simulink model "FOC_sensored"  (R2026a)
settings: Solver=VariableStepAuto  StopTime=0.5  MaxStep=1e-4  RelTol=1e-4
values from neighbouring files (symbols this model uses):
  Encoder_resolution = 4000    [FOC_sensored_script.m]
  In = 1    [FOC_sensored_script.m]
  J = 0.1e-4    (= 1e-05)    [FOC_sensored_script.m]
  Kr_cont_current = (2*omega_n*tau_q*zeta - 1) / K_q    [FOC_sensored_script.m]
  Kr_cont_speed = (2*omega_n_speed*tau_w*zeta_speed - 1) / K_w    [FOC_sensored_script.m]
  Kr_direct_back_current = (1-delta2*exp(Ts_current/tau_q)) / (K_q*(exp(Ts_current/tau_q)-1))    [FOC_sensored_script.m]
  Kr_direct_back_speed = (1-delta2*exp(Ts_speed/tau_w)) / (K_w*(exp(Ts_speed/tau_w)-1))    [FOC_sensored_script.m]
  Kr_direct_forw_current = (1+(1+delta1)*exp(Ts_current/tau_q)) / (K_q*(exp(Ts_current/tau_q)-1))    [FOC_sensored_script.m]
  Kr_direct_tustin_current = (2-exp(Ts_current/tau_q)*(delta2-delta1-1)) / (2*K_q*(exp(Ts_current/tau_q)-1))    [FOC_sensored_script.m]
  Kr_direct_tustin_speed = (2-exp(Ts_speed/tau_w)*(delta2-delta1-1)) / (2*K_w*(exp(Ts_speed/tau_w)-1))    [FOC_sensored_script.m]
  Ls = 330e-6/2    (= 0.000165)    [FOC_sensored_script.m]
  Mn = Pn/wn    [FOC_sensored_script.m]
  nn = ns/pp    (= 6000)    [FOC_sensored_script.m]
  pp = (60*fs)/ns    (= 4)    [FOC_sensored_script.m]
  Psir = 0.0064    [FOC_sensored_script.m]
  T_speed_feedback = 0.0005    [FOC_sensored_script.m]
  Ti_cont_current = (2*omega_n*tau_q*zeta - 1) / (tau_q * omega_n^2)    [FOC_sensored_script.m]
  Ti_cont_speed = (2*omega_n_speed*tau_w*zeta_speed - 1) / (tau_w * omega_n_speed^2)    [FOC_sensored_script.m]
  Ti_direct_back_current = Ts_current * (exp(-Ts_current/tau_q)-delta2) / (1+delta1+delta2)    [FOC_sensored_script.m]
  Ti_direct_back_speed = Ts_speed * (exp(-Ts_speed/tau_w)-delta2) / (1+delta1+delta2)    [FOC_sensored_script.m]
  Ti_direct_forw_current = Ts_current * (1+delta1+exp(-Ts_current/tau_q)) / (1+delta1+delta2)    [FOC_sensored_script.m]
  Ti_direct_forw_speed = Ts_speed * (1+delta1+exp(-Ts_speed/tau_w)) / (1+delta1+delta2)    [FOC_sensored_script.m]
  Ti_direct_tustin_current = Ts_current*(2*exp(-Ts_current/tau_q)+delta1-delta2+1) / (2*(1+delta1+delta2))    [FOC_sensored_script.m]
  Ti_direct_tustin_speed = Ts_speed*(2*exp(-Ts_speed/tau_w)+delta1-delta2+1) / (2*(1+delta1+delta2))    [FOC_sensored_script.m]
  Ts_current = 100e-6    (= 0.0001)    [FOC_sensored_script.m]
  Udc = 24    [FOC_sensored_script.m]
undefined symbols (not defined in the file or in its folder): Ld, Lq
libraries: fl_lib x48, nesl_utility x42, ee_lib x18, eeTransforms x12
(part 3 of 3)

== system FOC_sensored/PWM inverter7 ==
  ud_ref : Inport
  uq_ref : Inport  Port=2
  theta_e_mj : Inport  Port=3
  Constant1 : Constant  Value=0  SampleTime=-1
  Gain : Gain
  Gain1 : Gain
  Mux2 : Mux  Inputs=2
  Mux3 : Mux  Inputs=2
  Scope : Scope  NumInputPorts=2
      settings: ActiveDisplayYMinimum=-5.00439749396322  ActiveDisplayYMaximum=16.069405098335697
  Zero-Order Hold1 : ZeroOrderHold  SampleTime=Ts_current
  dq->abc : eeTransforms/Inverse Park Transform  AxisAlignment=D-axis  PowerInvariant=off
  u_abc* : Outport  VectorParamsAs1DForOutWhenUnconnected=off
  wires:
  Constant1/1 -> Mux2/2
  Mux2/1 -> dq->abc/1
  Mux3/1 -> Mux2/1
  theta_e_mj/1 -> dq->abc/2
  dq->abc/1 -> Zero-Order Hold1/1
  ud_ref/1 -> Gain/1
  uq_ref/1 -> Gain1/1
  Gain/1 -> Scope/1, Mux3/1
  Gain1/1 -> Scope/2, Mux3/2
  Zero-Order Hold1/1 -> u_abc*/1

== matlab function FOC_sensored/Low-Pass Filter Speed ==
  data: x input; y output; y_prev input; y_prev_out output; x_prev input; x_prev_out output; fc input; TS input
function [y, y_prev_out, x_prev_out] = fcn(x, y_prev, x_prev, fc, TS)


%% Convert to rad/s
omega_c = 2 * pi * fc;

%% Tustin coefficients
b =  omega_c / (2/TS + omega_c);
a = (omega_c - 2/TS) / (2/TS + omega_c);

%% Output
y = b * (x + x_prev) - a * y_prev;

%% State outputs — two separate scalars
y_prev_out = y;
x_prev_out = x;

end

== matlab function FOC_sensored/Low-Pass Filter Current ==
  data: x input; y output; y_prev input; y_prev_out output; x_prev input; x_prev_out output; fc input; TS input
function [y, y_prev_out, x_prev_out] = fcn(x, y_prev, x_prev, fc, TS)



%% Convert to rad/s
omega_c = 2 * pi * fc;

%% Tustin coefficients
b =  omega_c / (2/TS + omega_c);
a = (omega_c - 2/TS) / (2/TS + omega_c);

%% Output
y = b * (x + x_prev) - a * y_prev;

%% State outputs — two separate scalars
y_prev_out = y;
x_prev_out = x;

end

== matlab function FOC_sensored/Low-Pass Filter Speed Ref ==
  data: x input; y output; y_prev input; y_prev_out output; x_prev input; x_prev_out output; fc input; TS input
function [y, y_prev_out, x_prev_out] = fcn(x, y_prev, x_prev, fc, TS)

%% Convert to rad/s
omega_c = 2 * pi * fc;

%% Tustin coefficients
b =  omega_c / (2/TS + omega_c);
a = (omega_c - 2/TS) / (2/TS + omega_c);

%% Output
y = b * (x + x_prev) - a * y_prev;

%% State outputs — two separate scalars
y_prev_out = y;
x_prev_out = x;

end

== matlab function FOC_sensored/Diskretni regulator brzine1/PI-speed_controller ==
  data: speed_ref input; is_ref output; speed input; error_prev input; integrator_state input; error_out output; vd_state_out output; speed_ref_sat output; MAX_RPM input; K_P_speed input; K_I_speed input; TS input; IS_REF_LIMIT input
function [is_ref, error_out, vd_state_out,speed_ref_sat] = ...
          fcn(speed_ref, speed, error_prev, integrator_state, MAX_RPM, K_P_speed, K_I_speed, TS, IS_REF_LIMIT)



%% Saturate speed reference
if speed_ref > MAX_RPM
    speed_ref_sat = MAX_RPM;
elseif speed_ref < -MAX_RPM
    speed_ref_sat = -MAX_RPM;
else
    speed_ref_sat = speed_ref;
end

%% Error
error_curr = speed_ref_sat - speed;

%% --- Tustin (bilinear) PI ---
%
%  Continuous PI:   u(s) = Kp * e(s) + Ki/s * e(s)
%
%  Tustin:  integrator  1/s  ->  T/2 * (z+1)/(z-1)
%
%  Incremental form:
%    u[k] = u[k-1] + Kp*(e[k] - e[k-1]) + Ki*T/2*(e[k] + e[k-1])

is_ref_raw = integrator_state ...
           + K_P_speed * (error_curr - error_prev) ...
           + K_I_speed * (TS / 2.0) * (error_curr + error_prev);

%% Saturate is_ref (anti-windup: clamp before feeding state back)
if is_ref_raw > IS_REF_LIMIT
    is_ref = IS_REF_LIMIT;
elseif is_ref_raw < -IS_REF_LIMIT
    is_ref = -IS_REF_LIMIT;
else
    is_ref = is_ref_raw;
end

%% State outputs → Unit Delays → next step inputs
error_out      = error_curr;   % → Unit Delay → error_prev
vd_state_out   = is_ref;       % → Unit Delay → integrator_state (clamped = anti-windup)

end

== matlab function FOC_sensored/Diskretni regulatori struje2/PI-controller ==
  data: error_id input; error_iq input; id input; iq input; we_prev input; vd output; vq output; vd_state_in input; vq_state_in input; error_id_prev input; error_iq_prev input; vd_state_out output; vq_state_out output; error_id_out output; error_iq_out output; ff_id_prev input; ff_iq_prev input; ff_id_out output; ff_iq_out output; K_P_current input; K_I_current input; TS input; L_Q input; L_D input; PHI_PM input; CURRENT_CONTROL_LIMIT input
function [vd, vq, vd_state_out, vq_state_out, ...
          error_id_out, error_iq_out, ff_id_out, ff_iq_out] = ...
          fcn(error_id, error_iq, id, iq, we_prev, ...
              vd_state_in, vq_state_in, ...
              error_id_prev, error_iq_prev, ...
              ff_id_prev, ff_iq_prev, K_P_current, K_I_current, TS, L_Q, L_D, PHI_PM, CURRENT_CONTROL_LIMIT)


%% Feedforward — using delayed we to break algebraic loop
ff_id = -iq * L_Q * we_prev;
ff_iq =  id * L_D * we_prev + PHI_PM * we_prev;

%% Tustin PI + FF delta
vd_ = vd_state_in ...
    + K_P_current * (error_id - error_id_prev) ...
    + K_I_current * (TS / 2) * (error_id + error_id_prev) ...
    + (ff_id - ff_id_prev);

vq_ = vq_state_in ...
    + K_P_current * (error_iq - error_iq_prev) ...
    + K_I_current * (TS / 2) * (error_iq + error_iq_prev) ...
    + (ff_iq - ff_iq_prev);

%% Circle clamp
voltage_magnitude = sqrt(vd_^2 + vq_^2);
if voltage_magnitude > CURRENT_CONTROL_LIMIT
    scale = CURRENT_CONTROL_LIMIT / voltage_magnitude;
    vd = vd_ * scale;
    vq = vq_ * scale;
else
    vd = vd_;
    vq = vq_;
end

%% State outputs
vd_state_out = vd;
vq_state_out = vq;
error_id_out = error_id;
error_iq_out = error_iq;
ff_id_out    = ff_id;      % → Unit Delay → ff_id_prev
ff_iq_out    = ff_iq;      % → Unit Delay → ff_iq_prev

end

== matlab function FOC_sensored/Encoder1 ==
  data: angle input; theta_e output; omega_e output; angle_prev input; q_angle output; N input; dt input; pole_pairs input
function [theta_e, omega_e, q_angle] = fcn(angle, angle_prev, N, dt, pole_pairs)

%% Quantize current angle (simulate encoder resolution)
raw_count   = angle * (N / (2*pi));
counts      = floor(raw_count + 0.5);
q_angle     = counts * (2*pi / N);

%% Quantize previous angle the same way
raw_count_prev = angle_prev * (N / (2*pi));
counts_prev    = floor(raw_count_prev + 0.5);
q_angle_prev   = counts_prev * (2*pi / N);

%% Mechanical angular velocity (handle wrap-around)
delta = q_angle - q_angle_prev;

% Unwrap: if jump > pi, crossed zero boundary
if delta > pi
    delta = delta - 2*pi;
elseif delta < -pi
    delta = delta + 2*pi;
end

omega_m = delta / dt;       % mechanical rad/s

%% Convert to electrical quantities
theta_e = mod(q_angle, 2*pi);   % electrical angle [0, 2pi]
omega_e = omega_m;               % electrical rad/s

end

== matlab function FOC_sensored/Low-Pass Filter Current1 ==
  data: x input; y output; y_prev input; y_prev_out output; x_prev input; x_prev_out output; fc input; TS input
function [y, y_prev_out, x_prev_out] = fcn(x, y_prev, x_prev, fc, TS)



%% Convert to rad/s
omega_c = 2 * pi * fc;

%% Tustin coefficients
b =  omega_c / (2/TS + omega_c);
a = (omega_c - 2/TS) / (2/TS + omega_c);

%% Output
y = b * (x + x_prev) - a * y_prev;

%% State outputs — two separate scalars
y_prev_out = y;
x_prev_out = x;

end

== matlab function FOC_sensored/Low-Pass Filter Speed Ref1 ==
  data: x input; y output; y_prev input; y_prev_out output; x_prev input; x_prev_out output; fc input; TS input
function [y, y_prev_out, x_prev_out] = fcn(x, y_prev, x_prev, fc, TS)

%% Convert to rad/s
omega_c = 2 * pi * fc;

%% Tustin coefficients
b =  omega_c / (2/TS + omega_c);
a = (omega_c - 2/TS) / (2/TS + omega_c);

%% Output
y = b * (x + x_prev) - a * y_prev;

%% State outputs — two separate scalars
y_prev_out = y;
x_prev_out = x;

end

== matlab function FOC_sensored/Low-Pass Filter Speed1 ==
  data: x input; y output; y_prev input; y_prev_out output; x_prev input; x_prev_out output; fc input; TS input
function [y, y_prev_out, x_prev_out] = fcn(x, y_prev, x_prev, fc, TS)


%% Convert to rad/s
omega_c = 2 * pi * fc;

%% Tustin coefficients
b =  omega_c / (2/TS + omega_c);
a = (omega_c - 2/TS) / (2/TS + omega_c);

%% Output
y = b * (x + x_prev) - a * y_prev;

%% State outputs — two separate scalars
y_prev_out = y;
x_prev_out = x;

end

== matlab function FOC_sensored/Diskretni regulator brzine2/PI-speed_controller ==
  data: speed_ref input; is_ref output; vd_state_out output; speed input; vd_state_in input; error_prev input; error_out output; MAX_RPM input; K_P_speed input; K_I_speed input; TS input; IS_REF_LIMIT input
function [is_ref, vd_state_out, error_out] = ...
          fcn(speed_ref, speed, vd_state_in, error_prev, MAX_RPM, K_P_speed, K_I_speed, TS, IS_REF_LIMIT)


%% Saturate speed reference
if speed_ref > MAX_RPM
    speed_ref_sat = MAX_RPM;
elseif speed_ref < -MAX_RPM
    speed_ref_sat = -MAX_RPM;
else
    speed_ref_sat = speed_ref;
end

%% Error
error_curr = speed_ref_sat - speed;

%% --- Backward Euler PI ---
%
%  u[k] = u[k-1] + Kp*(e[k] - e[k-1]) + Ki*TS*e[k]

is_ref_raw = vd_state_in ...
           + K_P_speed * (error_curr - error_prev) ...
           + K_I_speed * TS * error_curr;

%% Saturate is_ref
if is_ref_raw > IS_REF_LIMIT
    is_ref = IS_REF_LIMIT;
elseif is_ref_raw < -IS_REF_LIMIT
    is_ref = -IS_REF_LIMIT;
else
    is_ref = is_ref_raw;
end

%% Conditional anti-windup — freeze integrator when saturated
saturated = (is_ref_raw > IS_REF_LIMIT && error_curr > 0) || ...
            (is_ref_raw < -IS_REF_LIMIT && error_curr < 0);

if saturated
    vd_state_out = vd_state_in;   % freeze
else
    vd_state_out = is_ref;
end

%% State output
error_out = error_curr;

end

== matlab function FOC_sensored/Diskretni regulatori struje1/PI-controller ==
  data: error_id input; error_iq input; vd output; vq output; vd_state_in input; vq_state_in input; vd_state_out output; vq_state_out output; error_id_prev input; error_iq_prev input; error_id_out output; error_iq_out output; K_P_current input; K_I_current input; TS input; CURRENT_CONTROL_LIMIT input
function [vd, vq, vd_state_out, vq_state_out, ...
          error_id_out, error_iq_out] = ...
          fcn(error_id, error_iq, ...
              vd_state_in, vq_state_in, ...
              error_id_prev, error_iq_prev, K_P_current, K_I_current, TS, CURRENT_CONTROL_LIMIT)


%% Backward Euler PI — incremental form
%
%  u[k] = u[k-1] + Kp*(e[k] - e[k-1]) + Ki*TS*e[k]

vd_ = vd_state_in ...
    + K_P_current * (error_id - error_id_prev) ...
    + K_I_current * TS * error_id;

vq_ = vq_state_in ...
    + K_P_current * (error_iq - error_iq_prev) ...
    + K_I_current * TS * error_iq;

%% Circle clamp
voltage_magnitude = sqrt(vd_^2 + vq_^2);
if voltage_magnitude > CURRENT_CONTROL_LIMIT
    scale = CURRENT_CONTROL_LIMIT / voltage_magnitude;
    vd = vd_ * scale;
    vq = vq_ * scale;
else
    vd = vd_;
    vq = vq_;
end

%% State outputs
vd_state_out  = vd;     % anti-windup: feed back clamped value
vq_state_out  = vq;
error_id_out  = error_id;
error_iq_out  = error_iq;

end

== matlab function FOC_sensored/Encoder2 ==
  data: angle input; theta_e output; omega_e output; angle_prev input; q_angle output; N input; dt input; pole_pairs input
function [theta_e, omega_e, q_angle] = fcn(angle, angle_prev, N, dt, pole_pairs)

%% Quantize current angle (simulate encoder resolution)
raw_count   = angle * (N / (2*pi));
counts      = floor(raw_count + 0.5);
q_angle     = counts * (2*pi / N);

%% Quantize previous angle the same way
raw_count_prev = angle_prev * (N / (2*pi));
counts_prev    = floor(raw_count_prev + 0.5);
q_angle_prev   = counts_prev * (2*pi / N);

%% Mechanical angular velocity (handle wrap-around)
delta = q_angle - q_angle_prev;

% Unwrap: if jump > pi, crossed zero boundary
if delta > pi
    delta = delta - 2*pi;
elseif delta < -pi
    delta = delta + 2*pi;
end

omega_m = delta / dt;       % mechanical rad/s

%% Convert to electrical quantities
theta_e = mod(q_angle, 2*pi);   % electrical angle [0, 2pi]
omega_e = omega_m;               % electrical rad/s

end

== matlab function FOC_sensored/Low-Pass Filter Current2 ==
  data: x input; y output; y_prev input; y_prev_out output; fc input; TS input
function [y, y_prev_out] = fcn(x, y_prev, fc, TS)


%% Convert to rad/s
omega_c = 2 * pi * fc;

%% Backward Euler discretization of H(s) = omega_c / (s + omega_c)
%
%  Backward Euler:  s -> (z-1)/(TS*z)
%
%  H(z) = omega_c / ((z-1)/(TS*z) + omega_c)
%
%  Multiply numerator and denominator by TS*z:
%
%  H(z) = omega_c*TS*z / ((z-1) + omega_c*TS*z)
%
%  Collecting z terms:
%
%  numerator:   omega_c*TS * z
%  denominator: (1 + omega_c*TS)*z - 1
%
%  Divide by (1 + omega_c*TS):
%
%  b = omega_c*TS / (1 + omega_c*TS)
%  a = 1 / (1 + omega_c*TS)
%
%  Difference equation:
%  y[k] = b*x[k] + a*y[k-1]

%% Precompute coefficients
b = (omega_c*TS) / (1 + omega_c*TS);
a = 1 / (1 + omega_c*TS);

%% Output — note: Backward Euler only needs y_prev, not x_prev
y = b * x + a * y_prev;

%% State outputs
y_prev_out = y;

end

== matlab function FOC_sensored/Low-Pass Filter Speed Ref2 ==
  data: x input; y output; y_prev input; y_prev_out output; fc input; TS input
function [y, y_prev_out] = fcn(x, y_prev, fc, TS)


%% Convert to rad/s
omega_c = 2 * pi * fc;

%% Backward Euler discretization of H(s) = omega_c / (s + omega_c)
%
%  Backward Euler:  s -> (z-1)/(TS*z)
%
%  H(z) = omega_c / ((z-1)/(TS*z) + omega_c)
%
%  Multiply numerator and denominator by TS*z:
%
%  H(z) = omega_c*TS*z / ((z-1) + omega_c*TS*z)
%
%  Collecting z terms:
%
%  numerator:   omega_c*TS * z
%  denominator: (1 + omega_c*TS)*z - 1
%
%  Divide by (1 + omega_c*TS):
%
%  b = omega_c*TS / (1 + omega_c*TS)
%  a = 1 / (1 + omega_c*TS)
%
%  Difference equation:
%  y[k] = b*x[k] + a*y[k-1]

%% Precompute coefficients
b = (omega_c*TS) / (1 + omega_c*TS);
a = 1 / (1 + omega_c*TS);

%% Output — note: Backward Euler only needs y_prev, not x_prev
y = b * x + a * y_prev;

%% State outputs
y_prev_out = y;

end

== matlab function FOC_sensored/Low-Pass Filter Speed2 ==
  data: x input; y output; y_prev input; y_prev_out output; fc input; TS input
function [y, y_prev_out] = fcn(x, y_prev, fc, TS)


%% Convert to rad/s
omega_c = 2 * pi * fc;

%% Backward Euler discretization of H(s) = omega_c / (s + omega_c)
%
%  Backward Euler:  s -> (z-1)/(TS*z)
%
%  H(z) = omega_c / ((z-1)/(TS*z) + omega_c)
%
%  Multiply numerator and denominator by TS*z:
%
%  H(z) = omega_c*TS*z / ((z-1) + omega_c*TS*z)
%
%  Collecting z terms:
%
%  numerator:   omega_c*TS * z
%  denominator: (1 + omega_c*TS)*z - 1
%
%  Divide by (1 + omega_c*TS):
%
%  b = omega_c*TS / (1 + omega_c*TS)
%  a = 1 / (1 + omega_c*TS)
%
%  Difference equation:
%  y[k] = b*x[k] + a*y[k-1]

%% Precompute coefficients
b = (omega_c*TS) / (1 + omega_c*TS);
a = 1 / (1 + omega_c*TS);

%% Output — note: Backward Euler only needs y_prev, not x_prev
y = b * x + a * y_prev;

%% State outputs
y_prev_out = y;

end

== matlab function FOC_sensored/Diskretni regulator brzine3/PI-speed_controller ==
  data: speed_ref input; is_ref output; speed input; error_prev input; integrator_state input; error_out output; vd_state_out output; speed_ref_sat output; MAX_RPM input; K_P_speed input; K_I_speed input; TS input; IS_REF_LIMIT input
function [is_ref, error_out, vd_state_out,speed_ref_sat] = ...
          fcn(speed_ref, speed, error_prev, integrator_state, MAX_RPM, K_P_speed, K_I_speed, TS, IS_REF_LIMIT)



%% Saturate speed reference
if speed_ref > MAX_RPM
    speed_ref_sat = MAX_RPM;
elseif speed_ref < -MAX_RPM
    speed_ref_sat = -MAX_RPM;
else
    speed_ref_sat = speed_ref;
end

%% Error
error_curr = speed_ref_sat - speed;

%% --- Tustin (bilinear) PI ---
%
%  Continuous PI:   u(s) = Kp * e(s) + Ki/s * e(s)
%
%  Tustin:  integrator  1/s  ->  T/2 * (z+1)/(z-1)
%
%  Incremental form:
%    u[k] = u[k-1] + Kp*(e[k] - e[k-1]) + Ki*T/2*(e[k] + e[k-1])

is_ref_raw = integrator_state ...
           + K_P_speed * (error_curr - error_prev) ...
           + K_I_speed * (TS / 2.0) * (error_curr + error_prev);

%% Saturate is_ref (anti-windup: clamp before feeding state back)
if is_ref_raw > IS_REF_LIMIT
    is_ref = IS_REF_LIMIT;
elseif is_ref_raw < -IS_REF_LIMIT
    is_ref = -IS_REF_LIMIT;
else
    is_ref = is_ref_raw;
end

%% State outputs → Unit Delays → next step inputs
error_out      = error_curr;   % → Unit Delay → error_prev
vd_state_out   = is_ref;       % → Unit Delay → integrator_state (clamped = anti-windup)

end

== matlab function FOC_sensored/Diskretni regulatori struje3/PI-controller ==
  data: error_id input; error_iq input; id input; iq input; we_prev input; vd output; vq output; vd_state_in input; vq_state_in input; error_id_prev input; error_iq_prev input; vd_state_out output; vq_state_out output; error_id_out output; error_iq_out output; ff_id_prev input; ff_iq_prev input; ff_id_out output; ff_iq_out output; K_P_current input; K_I_current input; TS input; L_Q input; L_D input; PHI_PM input; CURRENT_CONTROL_LIMIT input
function [vd, vq, vd_state_out, vq_state_out, ...
          error_id_out, error_iq_out, ff_id_out, ff_iq_out] = ...
          fcn(error_id, error_iq, id, iq, we_prev, ...
              vd_state_in, vq_state_in, ...
              error_id_prev, error_iq_prev, ...
              ff_id_prev, ff_iq_prev, K_P_current, K_I_current, TS, L_Q, L_D, PHI_PM, CURRENT_CONTROL_LIMIT)


%% Feedforward — using delayed we to break algebraic loop
ff_id = -iq * L_Q * we_prev;
ff_iq =  id * L_D * we_prev + PHI_PM * we_prev;

%% Tustin PI + FF delta
vd_ = vd_state_in ...
    + K_P_current * (error_id - error_id_prev) ...
    + K_I_current * (TS / 2) * (error_id + error_id_prev) ...
    + (ff_id - ff_id_prev);

vq_ = vq_state_in ...
    + K_P_current * (error_iq - error_iq_prev) ...
    + K_I_current * (TS / 2) * (error_iq + error_iq_prev) ...
    + (ff_iq - ff_iq_prev);

%% Circle clamp
voltage_magnitude = sqrt(vd_^2 + vq_^2);
if voltage_magnitude > CURRENT_CONTROL_LIMIT
    scale = CURRENT_CONTROL_LIMIT / voltage_magnitude;
    vd = vd_ * scale;
    vq = vq_ * scale;
else
    vd = vd_;
    vq = vq_;
end

%% State outputs
vd_state_out = vd;
vq_state_out = vq;
error_id_out = error_id;
error_iq_out = error_iq;
ff_id_out    = ff_id;      % → Unit Delay → ff_id_prev
ff_iq_out    = ff_iq;      % → Unit Delay → ff_iq_prev

end

== matlab function FOC_sensored/Encoder3 ==
  data: angle input; theta_e output; omega_e output; angle_prev input; q_angle output; N input; dt input; pole_pairs input
function [theta_e, omega_e, q_angle] = fcn(angle, angle_prev, N, dt, pole_pairs)

%% Quantize current angle (simulate encoder resolution)
raw_count   = angle * (N / (2*pi));
counts      = floor(raw_count + 0.5);
q_angle     = counts * (2*pi / N);

%% Quantize previous angle the same way
raw_count_prev = angle_prev * (N / (2*pi));
counts_prev    = floor(raw_count_prev + 0.5);
q_angle_prev   = counts_prev * (2*pi / N);

%% Mechanical angular velocity (handle wrap-around)
delta = q_angle - q_angle_prev;

% Unwrap: if jump > pi, crossed zero boundary
if delta > pi
    delta = delta - 2*pi;
elseif delta < -pi
    delta = delta + 2*pi;
end

omega_m = delta / dt;       % mechanical rad/s

%% Convert to electrical quantities
theta_e = mod(q_angle, 2*pi);   % electrical angle [0, 2pi]
omega_e = omega_m;               % electrical rad/s

end

== matlab function FOC_sensored/Low-Pass Filter Current3 ==
  data: x input; y output; y_prev input; y_prev_out output; x_prev input; x_prev_out output; fc input; TS input
function [y, y_prev_out, x_prev_out] = fcn(x, y_prev, x_prev, fc, TS)



%% Convert to rad/s
omega_c = 2 * pi * fc;

%% Tustin coefficients
b =  omega_c / (2/TS + omega_c);
a = (omega_c - 2/TS) / (2/TS + omega_c);

%% Output
y = b * (x + x_prev) - a * y_prev;

%% State outputs — two separate scalars
y_prev_out = y;
x_prev_out = x;

end

== matlab function FOC_sensored/Low-Pass Filter Speed Ref3 ==
  data: x input; y output; y_prev input; y_prev_out output; x_prev input; x_prev_out output; fc input; TS input
function [y, y_prev_out, x_prev_out] = fcn(x, y_prev, x_prev, fc, TS)

%% Convert to rad/s
omega_c = 2 * pi * fc;

%% Tustin coefficients
b =  omega_c / (2/TS + omega_c);
a = (omega_c - 2/TS) / (2/TS + omega_c);

%% Output
y = b * (x + x_prev) - a * y_prev;

%% State outputs — two separate scalars
y_prev_out = y;
x_prev_out = x;

end

== matlab function FOC_sensored/Low-Pass Filter Speed3 ==
  data: x input; y output; y_prev input; y_prev_out output; x_prev input; x_prev_out output; fc input; TS input
function [y, y_prev_out, x_prev_out] = fcn(x, y_prev, x_prev, fc, TS)


%% Convert to rad/s
omega_c = 2 * pi * fc;

%% Tustin coefficients
b =  omega_c / (2/TS + omega_c);
a = (omega_c - 2/TS) / (2/TS + omega_c);

%% Output
y = b * (x + x_prev) - a * y_prev;

%% State outputs — two separate scalars
y_prev_out = y;
x_prev_out = x;

end

== matlab function FOC_sensored/Diskretni regulator brzine4/PI-speed_controller ==
  data: speed_ref input; is_ref output; vd_state_out output; speed input; vd_state_in input; error_prev input; error_out output; MAX_RPM input; K_P_speed input; K_I_speed input; TS input; IS_REF_LIMIT input
function [is_ref, vd_state_out, error_out] = ...
          fcn(speed_ref, speed, vd_state_in, error_prev, MAX_RPM, K_P_speed, K_I_speed, TS, IS_REF_LIMIT)


%% Saturate speed reference
if speed_ref > MAX_RPM
    speed_ref_sat = MAX_RPM;
elseif speed_ref < -MAX_RPM
    speed_ref_sat = -MAX_RPM;
else
    speed_ref_sat = speed_ref;
end

%% Error
error_curr = speed_ref_sat - speed;

%% --- Forward Euler PI ---
%
%  u[k] = u[k-1] + Kp*(e[k] - e[k-1]) + Ki*TS*e[k-1]

is_ref_raw = vd_state_in ...
           + K_P_speed * (error_curr - error_prev) ...
           + K_I_speed * TS * error_prev;

%% Saturate is_ref
if is_ref_raw > IS_REF_LIMIT
    is_ref = IS_REF_LIMIT;
elseif is_ref_raw < -IS_REF_LIMIT
    is_ref = -IS_REF_LIMIT;
else
    is_ref = is_ref_raw;
end

%% Conditional anti-windup — freeze integrator when saturated
saturated = (is_ref_raw > IS_REF_LIMIT && error_curr > 0) || ...
            (is_ref_raw < -IS_REF_LIMIT && error_curr < 0);

if saturated
    vd_state_out = vd_state_in;   % freeze
else
    vd_state_out = is_ref;
end

%% State output
error_out = error_curr;

end

== matlab function FOC_sensored/Diskretni regulatori struje4/PI-controller ==
  data: error_id input; error_iq input; vd output; vq output; vd_state_in input; vq_state_in input; vd_state_out output; vq_state_out output; error_id_prev input; error_iq_prev input; error_id_out output; error_iq_out output; K_P_current input; K_I_current input; TS input; CURRENT_CONTROL_LIMIT input
function [vd, vq, vd_state_out, vq_state_out, ...
          error_id_out, error_iq_out] = ...
          fcn(error_id, error_iq, ...
              vd_state_in, vq_state_in, ...
              error_id_prev, error_iq_prev, K_P_current, K_I_current, TS, CURRENT_CONTROL_LIMIT)


%% Forward Euler PI — incremental form
%
%  Continuous PI:  u(s) = Kp*e(s) + Ki/s * e(s)
%
%  Forward Euler integral:  integral[k] = integral[k-1] + TS*e[k-1]
%
%  Incremental form:
%    u[k] = u[k-1] + Kp*(e[k] - e[k-1]) + Ki*TS*e[k-1]
%
%  Note: integral term uses e[k-1], NOT e[k] — this is what makes
%  it "forward" (uses past error to step forward)

vd_ = vd_state_in ...
    + K_P_current * (error_id - error_id_prev) ...
    + K_I_current * TS * error_id_prev;

vq_ = vq_state_in ...
    + K_P_current * (error_iq - error_iq_prev) ...
    + K_I_current * TS * error_iq_prev;

%% Circle clamp
voltage_magnitude = sqrt(vd_^2 + vq_^2);
if voltage_magnitude > CURRENT_CONTROL_LIMIT
    scale = CURRENT_CONTROL_LIMIT / voltage_magnitude;
    vd = vd_ * scale;
    vq = vq_ * scale;
else
    vd = vd_;
    vq = vq_;
end

%% State outputs
vd_state_out  = vd;
vq_state_out  = vq;
error_id_out  = error_id;
error_iq_out  = error_iq;

end

== matlab function FOC_sensored/Encoder4 ==
  data: angle input; theta_e output; omega_e output; angle_prev input; q_angle output; N input; dt input; pole_pairs input
function [theta_e, omega_e, q_angle] = fcn(angle, angle_prev, N, dt, pole_pairs)

%% Quantize current angle (simulate encoder resolution)
raw_count   = angle * (N / (2*pi));
counts      = floor(raw_count + 0.5);
q_angle     = counts * (2*pi / N);

%% Quantize previous angle the same way
raw_count_prev = angle_prev * (N / (2*pi));
counts_prev    = floor(raw_count_prev + 0.5);
q_angle_prev   = counts_prev * (2*pi / N);

%% Mechanical angular velocity (handle wrap-around)
delta = q_angle - q_angle_prev;

% Unwrap: if jump > pi, crossed zero boundary
if delta > pi
    delta = delta - 2*pi;
elseif delta < -pi
    delta = delta + 2*pi;
end

omega_m = delta / dt;       % mechanical rad/s

%% Convert to electrical quantities
theta_e = mod(q_angle, 2*pi);   % electrical angle [0, 2pi]
omega_e = omega_m;               % electrical rad/s

end

== matlab function FOC_sensored/Low-Pass Filter Current4 ==
  data: x input; y output; y_prev input; x_prev input; y_prev_out output; fc input; TS input; x_prev_out output
function [y, y_prev_out, x_prev_out] = fcn(x, y_prev, x_prev, fc, TS)


%% Convert to rad/s
omega_c = 2 * pi * fc;

%% Forward Euler discretization of H(s) = omega_c / (s + omega_c)
%
%  Forward Euler:  s -> (z-1)/TS
%
%  H(z) = omega_c / ((z-1)/TS + omega_c)
%
%  Multiply numerator and denominator by TS:
%
%  H(z) = omega_c*TS / ((z-1) + omega_c*TS)
%
%  Collecting z terms:
%
%  numerator:   omega_c*TS
%  denominator: z + (omega_c*TS - 1)
%
%  Difference equation derivation from H(z) = Y(z)/X(z):
%
%  z*Y(z) + (omega_c*TS - 1)*Y(z) = omega_c*TS*X(z)
%  y[k+1] = (1 - omega_c*TS)*y[k] + omega_c*TS*x[k]
%
%  Shifting index back by one (k -> k-1):
%  y[k] = (1 - omega_c*TS)*y[k-1] + omega_c*TS*x[k-1]
%
%  Note: Forward Euler uses x[k-1], NOT x[k] — this is the key difference

%% Precompute coefficients
a = 1 - omega_c*TS;
b = omega_c*TS;

%% Output — uses x_prev, not x (this is what makes it "forward")
y = a * y_prev + b * x_prev;

%% State outputs
y_prev_out = y;
x_prev_out = x;

end

== matlab function FOC_sensored/Encoder ==
  data: angle input; theta_e output; omega_e output; angle_prev input; q_angle output; N input; dt input; pole_pairs input
function [theta_e, omega_e, q_angle] = fcn(angle, angle_prev, N, dt, pole_pairs)

%% Quantize current angle (simulate encoder resolution)
raw_count   = angle * (N / (2*pi));
counts      = floor(raw_count + 0.5);
q_angle     = counts * (2*pi / N);

%% Quantize previous angle the same way
raw_count_prev = angle_prev * (N / (2*pi));
counts_prev    = floor(raw_count_prev + 0.5);
q_angle_prev   = counts_prev * (2*pi / N);

%% Mechanical angular velocity (handle wrap-around)
delta = q_angle - q_angle_prev;

% Unwrap: if jump > pi, crossed zero boundary
if delta > pi
    delta = delta - 2*pi;
elseif delta < -pi
    delta = delta + 2*pi;
end

omega_m = delta / dt;       % mechanical rad/s

%% Convert to electrical quantities
theta_e = mod(q_angle, 2*pi);   % electrical angle [0, 2pi]
omega_e = omega_m;               % electrical rad/s

end

== matlab function FOC_sensored/Low-Pass Filter Speed Ref4 ==
  data: x input; y output; y_prev input; x_prev input; y_prev_out output; fc input; TS input; x_prev_out output
function [y, y_prev_out, x_prev_out] = fcn(x, y_prev, x_prev, fc, TS)


%% Convert to rad/s
omega_c = 2 * pi * fc;

%% Forward Euler discretization of H(s) = omega_c / (s + omega_c)
%
%  Forward Euler:  s -> (z-1)/TS
%
%  H(z) = omega_c / ((z-1)/TS + omega_c)
%
%  Multiply numerator and denominator by TS:
%
%  H(z) = omega_c*TS / ((z-1) + omega_c*TS)
%
%  Collecting z terms:
%
%  numerator:   omega_c*TS
%  denominator: z + (omega_c*TS - 1)
%
%  Difference equation derivation from H(z) = Y(z)/X(z):
%
%  z*Y(z) + (omega_c*TS - 1)*Y(z) = omega_c*TS*X(z)
%  y[k+1] = (1 - omega_c*TS)*y[k] + omega_c*TS*x[k]
%
%  Shifting index back by one (k -> k-1):
%  y[k] = (1 - omega_c*TS)*y[k-1] + omega_c*TS*x[k-1]
%
%  Note: Forward Euler uses x[k-1], NOT x[k] — this is the key difference

%% Precompute coefficients
a = 1 - omega_c*TS;
b = omega_c*TS;

%% Output — uses x_prev, not x (this is what makes it "forward")
y = a * y_prev + b * x_prev;

%% State outputs
y_prev_out = y;
x_prev_out = x;

end

== matlab function FOC_sensored/Low-Pass Filter Speed4 ==
  data: x input; y output; y_prev input; y_prev_out output; x_prev input; x_prev_out output; fc input; TS input
function [y, y_prev_out, x_prev_out] = fcn(x, y_prev, x_prev, fc, TS)


%% Convert to rad/s
omega_c = 2 * pi * fc;

%% Forward Euler discretization of H(s) = omega_c / (s + omega_c)
%
%  Forward Euler:  s -> (z-1)/TS
%
%  H(z) = omega_c / ((z-1)/TS + omega_c)
%
%  Multiply numerator and denominator by TS:
%
%  H(z) = omega_c*TS / ((z-1) + omega_c*TS)
%
%  Collecting z terms:
%
%  numerator:   omega_c*TS
%  denominator: z + (omega_c*TS - 1)
%
%  Difference equation derivation from H(z) = Y(z)/X(z):
%
%  z*Y(z) + (omega_c*TS - 1)*Y(z) = omega_c*TS*X(z)
%  y[k+1] = (1 - omega_c*TS)*y[k] + omega_c*TS*x[k]
%
%  Shifting index back by one (k -> k-1):
%  y[k] = (1 - omega_c*TS)*y[k-1] + omega_c*TS*x[k-1]
%
%  Note: Forward Euler uses x[k-1], NOT x[k] — this is the key difference

%% Precompute coefficients
a = 1 - omega_c*TS;
b = omega_c*TS;

%% Output — uses x_prev, not x (this is what makes it "forward")
y = a * y_prev + b * x_prev;

%% State outputs
y_prev_out = y;
x_prev_out = x;

end

== matlab function FOC_sensored/Diskretni regulator brzine6/PI-speed_controller ==
  data: speed_ref input; is_ref output; vd_state_out output; speed input; vd_state_in input; error_prev input; error_out output; MAX_RPM input; K_P_speed input; K_I_speed input; TS input; IS_REF_LIMIT input
function [is_ref, vd_state_out, error_out] = ...
          fcn(speed_ref, speed, vd_state_in, error_prev, MAX_RPM, K_P_speed, K_I_speed, TS, IS_REF_LIMIT)


%% Saturate speed reference
if speed_ref > MAX_RPM
    speed_ref_sat = MAX_RPM;
elseif speed_ref < -MAX_RPM
    speed_ref_sat = -MAX_RPM;
else
    speed_ref_sat = speed_ref;
end

%% Error
error_curr = speed_ref_sat - speed;

%% --- Forward Euler PI ---
%
%  u[k] = u[k-1] + Kp*(e[k] - e[k-1]) + Ki*TS*e[k-1]

is_ref_raw = vd_state_in ...
           + K_P_speed * (error_curr - error_prev) ...
           + K_I_speed * TS * error_prev;

%% Saturate is_ref
if is_ref_raw > IS_REF_LIMIT
    is_ref = IS_REF_LIMIT;
elseif is_ref_raw < -IS_REF_LIMIT
    is_ref = -IS_REF_LIMIT;
else
    is_ref = is_ref_raw;
end

%% Conditional anti-windup — freeze integrator when saturated
saturated = (is_ref_raw > IS_REF_LIMIT && error_curr > 0) || ...
            (is_ref_raw < -IS_REF_LIMIT && error_curr < 0);

if saturated
    vd_state_out = vd_state_in;   % freeze
else
    vd_state_out = is_ref;
end

%% State output
error_out = error_curr;

end

== matlab function FOC_sensored/Diskretni regulatori struje6/PI-controller ==
  data: error_id input; error_iq input; vd output; vq output; vd_state_in input; vq_state_in input; vd_state_out output; vq_state_out output; error_id_prev input; error_iq_prev input; error_id_out output; error_iq_out output; K_P_current input; K_I_current input; TS input; CURRENT_CONTROL_LIMIT input
function [vd, vq, vd_state_out, vq_state_out, ...
          error_id_out, error_iq_out] = ...
          fcn(error_id, error_iq, ...
              vd_state_in, vq_state_in, ...
              error_id_prev, error_iq_prev, K_P_current, K_I_current, TS, CURRENT_CONTROL_LIMIT)


%% Forward Euler PI — incremental form
%
%  Continuous PI:  u(s) = Kp*e(s) + Ki/s * e(s)
%
%  Forward Euler integral:  integral[k] = integral[k-1] + TS*e[k-1]
%
%  Incremental form:
%    u[k] = u[k-1] + Kp*(e[k] - e[k-1]) + Ki*TS*e[k-1]
%
%  Note: integral term uses e[k-1], NOT e[k] — this is what makes
%  it "forward" (uses past error to step forward)

vd_ = vd_state_in ...
    + K_P_current * (error_id - error_id_prev) ...
    + K_I_current * TS * error_id_prev;

vq_ = vq_state_in ...
    + K_P_current * (error_iq - error_iq_prev) ...
    + K_I_current * TS * error_iq_prev;

%% Circle clamp
voltage_magnitude = sqrt(vd_^2 + vq_^2);
if voltage_magnitude > CURRENT_CONTROL_LIMIT
    scale = CURRENT_CONTROL_LIMIT / voltage_magnitude;
    vd = vd_ * scale;
    vq = vq_ * scale;
else
    vd = vd_;
    vq = vq_;
end

%% State outputs
vd_state_out  = vd;
vq_state_out  = vq;
error_id_out  = error_id;
error_iq_out  = error_iq;

end

== matlab function FOC_sensored/Encoder5 ==
  data: angle input; theta_e output; omega_e output; angle_prev input; q_angle output; N input; dt input; pole_pairs input
function [theta_e, omega_e, q_angle] = fcn(angle, angle_prev, N, dt, pole_pairs)

%% Quantize current angle (simulate encoder resolution)
raw_count   = angle * (N / (2*pi));
counts      = floor(raw_count + 0.5);
q_angle     = counts * (2*pi / N);

%% Quantize previous angle the same way
raw_count_prev = angle_prev * (N / (2*pi));
counts_prev    = floor(raw_count_prev + 0.5);
q_angle_prev   = counts_prev * (2*pi / N);

%% Mechanical angular velocity (handle wrap-around)
delta = q_angle - q_angle_prev;

% Unwrap: if jump > pi, crossed zero boundary
if delta > pi
    delta = delta - 2*pi;
elseif delta < -pi
    delta = delta + 2*pi;
end

omega_m = delta / dt;       % mechanical rad/s

%% Convert to electrical quantities
theta_e = mod(q_angle, 2*pi);   % electrical angle [0, 2pi]
omega_e = omega_m;               % electrical rad/s

end

== matlab function FOC_sensored/Low-Pass Filter Current5 ==
  data: x input; y output; y_prev input; x_prev input; y_prev_out output; fc input; TS input; x_prev_out output
function [y, y_prev_out, x_prev_out] = fcn(x, y_prev, x_prev, fc, TS)


%% Convert to rad/s
omega_c = 2 * pi * fc;

%% Forward Euler discretization of H(s) = omega_c / (s + omega_c)
%
%  Forward Euler:  s -> (z-1)/TS
%
%  H(z) = omega_c / ((z-1)/TS + omega_c)
%
%  Multiply numerator and denominator by TS:
%
%  H(z) = omega_c*TS / ((z-1) + omega_c*TS)
%
%  Collecting z terms:
%
%  numerator:   omega_c*TS
%  denominator: z + (omega_c*TS - 1)
%
%  Difference equation derivation from H(z) = Y(z)/X(z):
%
%  z*Y(z) + (omega_c*TS - 1)*Y(z) = omega_c*TS*X(z)
%  y[k+1] = (1 - omega_c*TS)*y[k] + omega_c*TS*x[k]
%
%  Shifting index back by one (k -> k-1):
%  y[k] = (1 - omega_c*TS)*y[k-1] + omega_c*TS*x[k-1]
%
%  Note: Forward Euler uses x[k-1], NOT x[k] — this is the key difference

%% Precompute coefficients
a = 1 - omega_c*TS;
b = omega_c*TS;

%% Output — uses x_prev, not x (this is what makes it "forward")
y = a * y_prev + b * x_prev;

%% State outputs
y_prev_out = y;
x_prev_out = x;

end

== matlab function FOC_sensored/Low-Pass Filter Speed Ref5 ==
  data: x input; y output; y_prev input; x_prev input; y_prev_out output; fc input; TS input; x_prev_out output
function [y, y_prev_out, x_prev_out] = fcn(x, y_prev, x_prev, fc, TS)


%% Convert to rad/s
omega_c = 2 * pi * fc;

%% Forward Euler discretization of H(s) = omega_c / (s + omega_c)
%
%  Forward Euler:  s -> (z-1)/TS
%
%  H(z) = omega_c / ((z-1)/TS + omega_c)
%
%  Multiply numerator and denominator by TS:
%
%  H(z) = omega_c*TS / ((z-1) + omega_c*TS)
%
%  Collecting z terms:
%
%  numerator:   omega_c*TS
%  denominator: z + (omega_c*TS - 1)
%
%  Difference equation derivation from H(z) = Y(z)/X(z):
%
%  z*Y(z) + (omega_c*TS - 1)*Y(z) = omega_c*TS*X(z)
%  y[k+1] = (1 - omega_c*TS)*y[k] + omega_c*TS*x[k]
%
%  Shifting index back by one (k -> k-1):
%  y[k] = (1 - omega_c*TS)*y[k-1] + omega_c*TS*x[k-1]
%
%  Note: Forward Euler uses x[k-1], NOT x[k] — this is the key difference

%% Precompute coefficients
a = 1 - omega_c*TS;
b = omega_c*TS;

%% Output — uses x_prev, not x (this is what makes it "forward")
y = a * y_prev + b * x_prev;

%% State outputs
y_prev_out = y;
x_prev_out = x;

end

== matlab function FOC_sensored/Low-Pass Filter Speed5 ==
  data: x input; y output; y_prev input; y_prev_out output; x_prev input; x_prev_out output; fc input; TS input
function [y, y_prev_out, x_prev_out] = fcn(x, y_prev, x_prev, fc, TS)


%% Convert to rad/s
omega_c = 2 * pi * fc;

%% Forward Euler discretization of H(s) = omega_c / (s + omega_c)
%
%  Forward Euler:  s -> (z-1)/TS
%
%  H(z) = omega_c / ((z-1)/TS + omega_c)
%
%  Multiply numerator and denominator by TS:
%
%  H(z) = omega_c*TS / ((z-1) + omega_c*TS)
%
%  Collecting z terms:
%
%  numerator:   omega_c*TS
%  denominator: z + (omega_c*TS - 1)
%
%  Difference equation derivation from H(z) = Y(z)/X(z):
%
%  z*Y(z) + (omega_c*TS - 1)*Y(z) = omega_c*TS*X(z)
%  y[k+1] = (1 - omega_c*TS)*y[k] + omega_c*TS*x[k]
%
%  Shifting index back by one (k -> k-1):
%  y[k] = (1 - omega_c*TS)*y[k-1] + omega_c*TS*x[k-1]
%
%  Note: Forward Euler uses x[k-1], NOT x[k] — this is the key difference

%% Precompute coefficients
a = 1 - omega_c*TS;
b = omega_c*TS;

%% Output — uses x_prev, not x (this is what makes it "forward")
y = a * y_prev + b * x_prev;

%% State outputs
y_prev_out = y;
x_prev_out = x;

end

== matlab function FOC_sensored/Diskretni regulatori struje5/PI-controller ==
  data: error_id input; error_iq input; id input; iq input; we_prev input; vd output; vq output; vd_state_in input; vq_state_in input; error_id_prev input; error_iq_prev input; vd_state_out output; vq_state_out output; error_id_out output; error_iq_out output; ff_id_prev input; ff_iq_prev input; ff_id_out output; ff_iq_out output; K_P_current input; K_I_current input; TS input; L_Q input; L_D input; PHI_PM input; CURRENT_CONTROL_LIMIT input
function [vd, vq, vd_state_out, vq_state_out, ...
          error_id_out, error_iq_out, ff_id_out, ff_iq_out] = ...
          fcn(error_id, error_iq, id, iq, we_prev, ...
              vd_state_in, vq_state_in, ...
              error_id_prev, error_iq_prev, ...
              ff_id_prev, ff_iq_prev, K_P_current, K_I_current, TS, L_Q, L_D, PHI_PM, CURRENT_CONTROL_LIMIT)


%% Feedforward — using delayed we to break algebraic loop
ff_id = -iq * L_Q * we_prev;
ff_iq =  id * L_D * we_prev + PHI_PM * we_prev;

%% Tustin PI + FF delta
vd_ = vd_state_in ...
    + K_P_current * (error_id - error_id_prev) ...
    + K_I_current * (TS / 2) * (error_id + error_id_prev) ...
    + (ff_id - ff_id_prev);

vq_ = vq_state_in ...
    + K_P_current * (error_iq - error_iq_prev) ...
    + K_I_current * (TS / 2) * (error_iq + error_iq_prev) ...
    + (ff_iq - ff_iq_prev);

%% Circle clamp
voltage_magnitude = sqrt(vd_^2 + vq_^2);
if voltage_magnitude > CURRENT_CONTROL_LIMIT
    scale = CURRENT_CONTROL_LIMIT / voltage_magnitude;
    vd = vd_ * scale;
    vq = vq_ * scale;
else
    vd = vd_;
    vq = vq_;
end

%% State outputs
vd_state_out = vd;
vq_state_out = vq;
error_id_out = error_id;
error_iq_out = error_iq;
ff_id_out    = ff_id;      % → Unit Delay → ff_id_prev
ff_iq_out    = ff_iq;      % → Unit Delay → ff_iq_prev

end

== matlab function FOC_sensored/Diskretni regulator brzine5/PI-speed_controller ==
  data: speed_ref input; is_ref output; speed input; error_prev input; integrator_state input; error_out output; vd_state_out output; speed_ref_sat output; MAX_RPM input; K_P_speed input; K_I_speed input; TS input; IS_REF_LIMIT input
function [is_ref, error_out, vd_state_out,speed_ref_sat] = ...
          fcn(speed_ref, speed, error_prev, integrator_state, MAX_RPM, K_P_speed, K_I_speed, TS, IS_REF_LIMIT)



%% Saturate speed reference
if speed_ref > MAX_RPM
    speed_ref_sat = MAX_RPM;
elseif speed_ref < -MAX_RPM
    speed_ref_sat = -MAX_RPM;
else
    speed_ref_sat = speed_ref;
end

%% Error
error_curr = speed_ref_sat - speed;

%% --- Tustin (bilinear) PI ---
%
%  Continuous PI:   u(s) = Kp * e(s) + Ki/s * e(s)
%
%  Tustin:  integrator  1/s  ->  T/2 * (z+1)/(z-1)
%
%  Incremental form:
%    u[k] = u[k-1] + Kp*(e[k] - e[k-1]) + Ki*T/2*(e[k] + e[k-1])

is_ref_raw = integrator_state ...
           + K_P_speed * (error_curr - error_prev) ...
           + K_I_speed * (TS / 2.0) * (error_curr + error_prev);

%% Saturate is_ref (anti-windup: clamp before feeding state back)
if is_ref_raw > IS_REF_LIMIT
    is_ref = IS_REF_LIMIT;
elseif is_ref_raw < -IS_REF_LIMIT
    is_ref = -IS_REF_LIMIT;
else
    is_ref = is_ref_raw;
end

%% State outputs → Unit Delays → next step inputs
error_out      = error_curr;   % → Unit Delay → error_prev
vd_state_out   = is_ref;       % → Unit Delay → integrator_state (clamped = anti-windup)

end
